simulink library "AirWaterHeatPumpTL"  (R2025a)
settings: Solver=VariableStepAuto  StartTime=0.0  StopTime=10.0  RelTol=1e-3
libraries: fl_lib x13, AirWaterHeatPump_lib x1, SimscapeFluids_lib x1
settings Model: Creator=vikrants  LastModifiedBy=vikrants

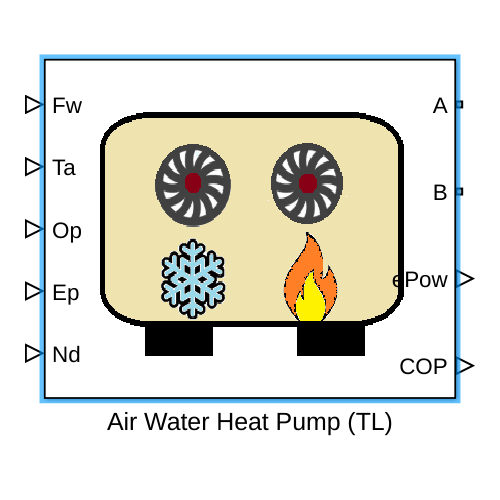
[thumbnail: Simulink's stored preview of the top-level diagram]
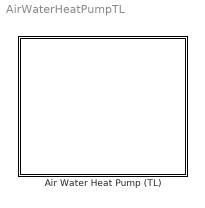
== system AirWaterHeatPumpTL ==
  Air Water Heat Pump (TL) : Subsystem  mask{heatingCapacityA=10.17, heatingCoPA=4.86, heatingCapacityB=10.12, heatingCoPB=3.7, heatingCapacityC=10.17, heatingCoPC=4.86, heatingCapacityD=10.12, heatingCoPD=3.7, coolingCapacityE=10.55, coolingCoPE=4.13, coolingCapacityF=6.9, coolingCoPF=2.7, elecHeaterPower=0, coilLen=2, coilArea=pi*(5e-2^2)/4, coilDia=5e-2, tankVolume=5, initialT=299.8, waterOpTempMax=330, waterOpTempMin=278, initialP=0.101325, measTimelagWater=60, minWaterFlowRate=1e-3, nomFlowDuringTest=0.5}
      mask prompts: heatingCapacityA "A-2W55, estimated heating capacity (kW)"; heatingCoPA "A-2W55, estimated COP (or SCOP)"; heatingCapacityB "A-2W65, estimated heating capacity (kW)"; heatingCoPB "A-2W65, estimated COP (or SCOP)"; heatingCapacityC "A7W35, estimated heating capacity (kW)"; heatingCoPC "A7W35, estimated COP (or SCOP)"; heatingCapacityD "A7W45, estimated heating capacity (kW)"; heatingCoPD "A7W45, estimated COP (or SCOP)"; coolingCapacityE "A35W18, estimated cooling capacity (kW)"; coolingCoPE "A35W18, estimated COP (or SCOP)"; coolingCapacityF "A35W7, estimated cooling capacity (kW)"; coolingCoPF "A35W7, estimated COP (or SCOP)"; elecHeaterPower "Additional electric heater rating (kW)"; coilLen "Length of coil pipe (m)"; coilArea "Area of coil pipe (m^2)"; coilDia "Diameter of coil pipe (m)"; tankVolume "Heat exchanger internal volume (m^3)"; initialT "Initial Temperature (K)"; waterOpTempMax "Maximum operational water temperature"; waterOpTempMin "Minimum operation water temperature"; initialP "Initial pressure of coil pipe water (MPa)"; measTimelagWater "Temperature sensor delay for water flow (s)"; minWaterFlowRate "Minimum water flowrate (kg/s)"; nomFlowDuringTest "Nominal water flowrate during test (kg/s)"
      mask Help: web("DocumentationAirWaterHeatPumpTL.html")
      mask DialogControl DescGroupVar Prompt: Description
      mask DialogControl DescTextVar Prompt: Heat pump model based on EN14511 test data.
      mask DialogControl Container3 Prompt: EN14511 (Heating) Data
      mask DialogControl Container4 Prompt: EN14511 (Cooling) Data
      mask DialogControl ParameterGroupVar Prompt: Heat Pump Construction
      mask DialogControl Container5 Prompt: Flow and Thermal Specifications
      mask Display: image('AirWaterHeatPumpTL.png');

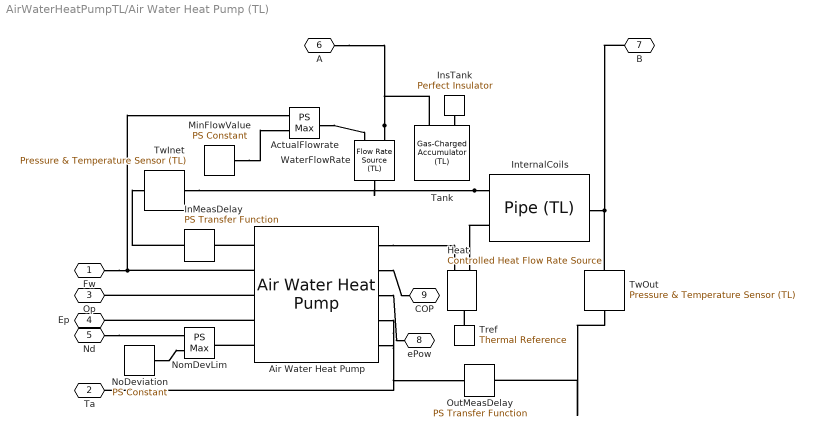
== system AirWaterHeatPumpTL/Air Water Heat Pump (TL) ==
  ActualFlowrate : fl_lib/Physical Signals/Nonlinear Operators/PS Max  ZeroCross=true
      settings: InternalSimscapePortConfiguration="{\"Bottom\":[],\"Left\":[{\"id\":\"I1\",\"label\":\"\",\"type\":\"input\"},{\"id\":\"I2\",\"label\":\"\",\"type\":\"input\"}],\"Right\":[{\"id\":\"O\",\"label\":\"\",\"type\":\"output\"}],\"Top\":[]}"
  Air Water Heat Pump : AirWaterHeatPump_lib/Air Water Heat Pump  nominalCapacityA=heatingCapacityA kW  seasonalCOPvalA=heatingCoPA  nominalCapacityB=heatingCapacityB kW  seasonalCOPvalB=heatingCoPB  nominalCapacityC=heatingCapacityC kW  seasonalCOPvalC=heatingCoPC  nominalCapacityD=heatingCapacityD kW  seasonalCOPvalD=heatingCoPD  nominalCapacityE=coolingCapacityE kW  seasonalCOPvalE=coolingCoPE  nominalCapacityF=coolingCapacityF kW  seasonalCOPvalF=coolingCoPF  backupElecHeater=elecHeaterPower kW  wInletOpRangeUpp=waterOpTempMax K  wInletOpRangeLow=waterOpTempMin K  airTemperatureVector=273 + [-2, -2, 7, 7, 35, 35]  waterTemperatureVector=273 + [55, 65, 35, 45, 18, 7]  waterSpHeat=4186 J/(K*kg)  smallPower=1e-3 W  maxCOP_specify=off  maxCOP_priority=None  maxCOP=8  maxCOP_nominal_specify=off  maxCOP_nominal_value=1  maxCOP_nominal_unit=1
      settings: InternalSimscapePortConfiguration="{\"Bottom\":[{\"id\":\"Ta\",\"label\":\"Ta\",\"type\":\"input\"},{\"id\":\"Tw\",\"label\":\"Tw\",\"type\":\"input\"}],\"Left\":[{\"id\":\"Tl\",\"label\":\"Tl\",\"type\":\"input\"},{\"id\":\"Fw\",\"label\":\"Fw\",\"type\":\"input\"},{\"id\":\"Op\",\"label\":\"Op\",\"type\":\"input\"},{\"id\":\"Ep\",\"label\":\"Ep\",\"type\":\"input\"},{\"id\":\"Nd\",\"label\":\"Nd\",\"type\":\"input\"}],\"Right\":[{\"id\":\"calcCap\",\"label\":\"Q\",\"type\":\"output\"},{\"id\":\"calcCOP\",\"label\":\"COP\",\"type\":\"output\"},{\"id\":\"ePower\",\"label\":\"ePow\",\"type\":\"output\"}],\"Top\":[]}"
  Heat : fl_lib/Thermal/Thermal Sources/Controlled Heat Flow Rate Source
  InMeasDelay : fl_lib/Physical Signals/Linear Operators/PS Transfer Function  transfer_function_type=foundation.enum.transfer_function_type.lag  T=measTimelagWater s  T1=2 s  T2=1 s  reset_method=foundation.enum.IntegratorResetSpec.None  initial_condition_spec=foundation.enum.IntegratorICSpec.Internal  y0=initialT K
      settings: InternalSimscapePortConfiguration="{\"Bottom\":[],\"Left\":[{\"id\":\"U\",\"label\":\"\",\"type\":\"input\"}],\"Right\":[{\"id\":\"Y\",\"label\":\"\",\"type\":\"output\"}],\"Top\":[]}"
  InsTank : fl_lib/Thermal/Thermal Elements/Perfect Insulator  T_specify=off  T_priority=None  T=293.15 K  T_nominal_specify=off  T_nominal_value=1  T_nominal_unit=K
  InternalCoils : fl_lib/Thermal Liquid/Elements/Pipe (TL)  length=coilLen m  area=coilArea m^2  Dh=coilDia m  length_add=0 m  roughness=15e-6 m  Re_lam=2000  Re_tur=4000  shape_factor=64  Nu_lam=3.66  dynamic_compressibility=true  inertia=false  p0=initialP MPa  T0=initialT K  mdot0=0 kg/s  p_nominal=0.101325 MPa  T_nominal=293.15 K
  MinFlowValue : fl_lib/Physical Signals/Sources/PS Constant  constant=minWaterFlowRate kg/s
  NoDeviation : fl_lib/Physical Signals/Sources/PS Constant  constant=1
  NomDevLim : fl_lib/Physical Signals/Nonlinear Operators/PS Max  ZeroCross=true
      settings: InternalSimscapePortConfiguration="{\"Bottom\":[],\"Left\":[{\"id\":\"I1\",\"label\":\"\",\"type\":\"input\"},{\"id\":\"I2\",\"label\":\"\",\"type\":\"input\"}],\"Right\":[{\"id\":\"O\",\"label\":\"\",\"type\":\"output\"}],\"Top\":[]}"
  OutMeasDelay : fl_lib/Physical Signals/Linear Operators/PS Transfer Function  transfer_function_type=foundation.enum.transfer_function_type.lag  T=measTimelagWater s  T1=2 s  T2=1 s  reset_method=foundation.enum.IntegratorResetSpec.None  initial_condition_spec=foundation.enum.IntegratorICSpec.Internal  y0=initialT K
      settings: InternalSimscapePortConfiguration="{\"Bottom\":[],\"Left\":[{\"id\":\"U\",\"label\":\"\",\"type\":\"input\"}],\"Right\":[{\"id\":\"Y\",\"label\":\"\",\"type\":\"output\"}],\"Top\":[]}"
  Tank : SimscapeFluids_lib/Thermal Liquid/Tanks & Accumulators/Gas-Charged Accumulator (TL)  capacity=tankVolume m^3  dead_volume=4e-5 m^3  p_precharge_gauge=0 MPa  k_sh=1.4  area=0.01 m^2  stiff_coeff=1e4 MPa/m^3  damping_coeff=1e4 MPa*s/m^6  liquid_volume_specify=off  liquid_volume_priority=High  liquid_volume=5e-3 m^3  liquid_volume_nominal_specify=off  liquid_volume_nominal_value=1  liquid_volume_nominal_unit=m^3  liquid_mass_specify=off  liquid_mass_priority=None  liquid_mass=5 kg  liquid_mass_nominal_specify=off  liquid_mass_nominal_value=1  liquid_mass_nominal_unit=kg  p_I_specify=off  p_I_priority=None  p_I=0.101325 MPa  p_I_nominal_specify=off  p_I_nominal_value=1  p_I_nominal_unit=MPa  T_I_specify=on  T_I_priority=High  T_I=initialT K  T_I_nominal_specify=off  T_I_nominal_value=1  T_I_nominal_unit=K
      settings: InternalSimscapePortConfiguration="{\"Bottom\":[],\"Left\":[],\"Right\":[{\"id\":\"A\",\"label\":\"A\",\"type\":\"foundation.thermal_liquid.thermal_liquid\"},{\"id\":\"H\",\"label\":\"H\",\"type\":\"foundation.thermal.thermal\"}],\"Top\":[]}"
  Tref : fl_lib/Thermal/Thermal Elements/Thermal Reference
  TwInet : fl_lib/Thermal Liquid/Sensors/Pressure & Temperature Sensor (TL)  reference=foundation.enum.MeasurementReference.absolute  pressure=false  pressure_spec=foundation.enum.PressureMeasementSpec.Absolute  temperature=true
      settings: InternalSimscapePortConfiguration="{\"Bottom\":[{\"id\":\"T\",\"label\":\"T\",\"type\":\"output\"}],\"Left\":[{\"id\":\"A\",\"label\":\"A\",\"type\":\"foundation.thermal_liquid.thermal_liquid\"}],\"Right\":[],\"Top\":[]}"
  TwOut : fl_lib/Thermal Liquid/Sensors/Pressure & Temperature Sensor (TL)  reference=foundation.enum.MeasurementReference.absolute  pressure=false  pressure_spec=foundation.enum.PressureMeasementSpec.Absolute  temperature=true
      settings: InternalSimscapePortConfiguration="{\"Bottom\":[{\"id\":\"T\",\"label\":\"T\",\"type\":\"output\"}],\"Left\":[{\"id\":\"A\",\"label\":\"A\",\"type\":\"foundation.thermal_liquid.thermal_liquid\"}],\"Right\":[],\"Top\":[]}"
  WaterFlowRate : fl_lib/Thermal Liquid/Sources/Flow Rate Source (TL)  source_type=foundation.enum.constant_controlled.controlled  flow_type=foundation.enum.mass_volumetric_flow.mass  mass_flow=0 kg/s  volumetric_flow=0 m^3/s  power_spec=foundation.enum.power_spec.none  area=coilArea m^2
  Fw : PMIOPort  Side=Left
  Ta : PMIOPort  Port=2  Side=Left
  Op : PMIOPort  Port=3  Side=Left
  Ep : PMIOPort  Port=4  Side=Left
  Nd : PMIOPort  Port=5  Side=Left
  A : PMIOPort  Port=6  Side=Right
  B : PMIOPort  Port=7  Side=Right
  ePow : PMIOPort  Port=8  Side=Right
  COP : PMIOPort  Port=9  Side=Right
  connections:
  TwOut/LConn1 -- B/RConn1 -- InternalCoils/RConn1
  InternalCoils/LConn1 -- WaterFlowRate/RConn1 -- TwInet/LConn1
  Fw/RConn1 -- Air Water Heat Pump/LConn2 -- ActualFlowrate/LConn1
  WaterFlowRate/LConn1 -- A/RConn1 -- Tank/RConn1
  Air Water Heat Pump/LConn1 -- InMeasDelay/RConn1
  Air Water Heat Pump/LConn3 -- Op/RConn1
  InMeasDelay/LConn1 -- TwInet/RConn1
  InternalCoils/LConn2 -- Heat/RConn2
  Air Water Heat Pump/RConn3 -- ePow/RConn1
  InsTank/LConn1 -- Tank/RConn2
  NoDeviation/RConn1 -- NomDevLim/LConn2
  Air Water Heat Pump/LConn4 -- Ep/RConn1
  Air Water Heat Pump/RConn2 -- COP/RConn1
  ActualFlowrate/RConn1 -- WaterFlowRate/LConn2
  MinFlowValue/RConn1 -- ActualFlowrate/LConn2
  Air Water Heat Pump/RConn5 -- OutMeasDelay/RConn1
  Tref/LConn1 -- Heat/LConn1
  Air Water Heat Pump/LConn5 -- NomDevLim/RConn1
  TwOut/RConn1 -- OutMeasDelay/LConn1
  Nd/RConn1 -- NomDevLim/LConn1
  Air Water Heat Pump/RConn4 -- Ta/RConn1
  Air Water Heat Pump/RConn1 -- Heat/RConn1
